simulink model "ebm_2022"  (R2022a)
settings: Solver=ode4  StartTime=0.0  StopTime=Inf  FixedStep=0.1  RelTol=1e-3  EnableMultiTasking=on
PreLoadFcn:
  | initialize;
values from neighbouring files (symbols this model uses):
  offset = 100.0*(mean(T_ambient) - mean(T_heater))    [initialize.m]
libraries: arduinolib x4, dspstat3 x2
PostSaveFcn:
  | initialize;
settings Model: ExtModeTrigDuration=2  Creator=user  LastModifiedBy=manur
settings SolverCC: AlgebraicLoopSolver=TrustRegion  AutoInsertRateTranBlk=on
settings DataIOCC: ReturnWorkspaceOutputs=off
settings OptimizationCC: EnhancedBackFolding=on  PassReuseOutputArgsAs=Individual arguments  MaxStackSize=64  OptimizeBlockOrder=speed  DifferentSizesBufferReuse=on  OptimizationCustomize=off  EfficientTunableParamExpr=on
settings DebuggingCC: ParameterTunabilityLossMsg=error  UnconnectedInputMsg=warning  UnconnectedOutputMsg=warning  UnconnectedLineMsg=warning  SFMachineParentedDataDiag=warning  ArithmeticOperatorsInVariantConditions=warning
settings HardwareCC: ProdBitPerInt=16  ProdBitPerPointer=16  ProdBitPerSizeT=16  ProdBitPerPtrDiffT=16  ProdLargestAtomicFloat=None  ProdWordSize=8  ProdHWDeviceType=Atmel->AVR
settings SFSimCC: SimUseLocalCustomCode=off  MATLABDynamicMemAlloc=off  CustomCodeUndefinedFunction=UseInterfaceOnly
settings SFSimCC: SimCustomInitializer=|
  | analogWrite(9, 255); // the fan has quite significant stiction friction, so we start with a full speed!
  | delay(10);
settings SFSimCC: SimCustomTerminator=|
  | analogWrite(9, 0);
  | analogWrite(10, 0);
  | delay(1);
settings RTWCC: SystemTargetFile=ert.tlc  HardwareBoard=Arduino Uno  TemplateMakefile=ert_default_tmf  GenerateReport=on  RTWUseLocalCustomCode=off  Toolchain=Arduino AVR  BuildConfiguration=Faster Runs  IncludeHyperlinkInReport=on  LaunchReport=on  GenerateTraceInfo=on  GenerateTraceReport=on  GenerateTraceReportSl=on  GenerateTraceReportSf=on  GenerateTraceReportEml=on  DLArmComputeVersion=19.05
settings CodeAppCC: ForceParamTrailComments=on  IgnoreCustomStorageClasses=off  OperatorAnnotations=on  SimulinkDataObjDesc=on  SFDataObjDesc=on  InsertBlockDesc=on
settings ERTTargetCC: SupportContinuousTime=on  SupportVariableSizeSignals=on  ExtMode=on  ExtModeMexArgs='127.0.0.1' 0 17725

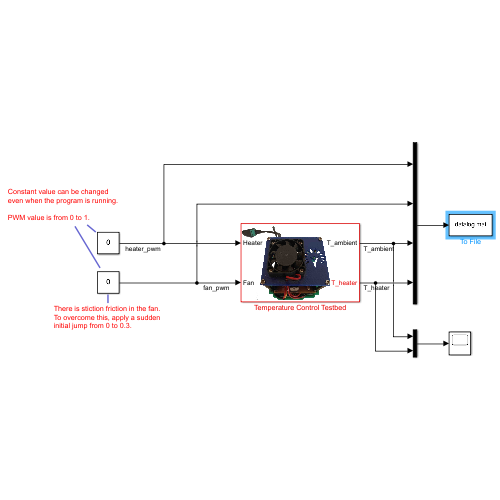
[thumbnail: Simulink's stored preview of the top-level diagram]
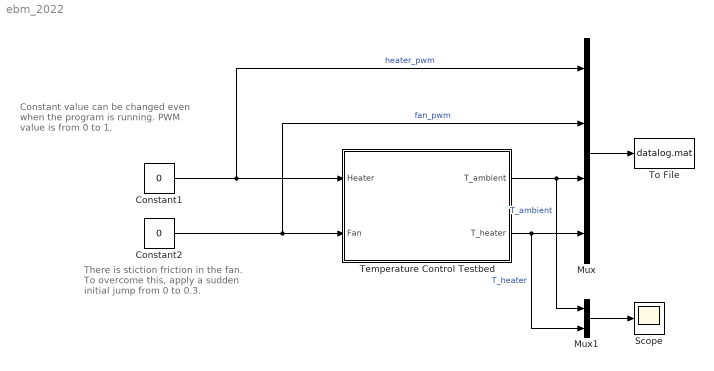
== system ebm_2022 ==
  note: There is stiction friction in the fan.
      | To overcome this, apply a sudden
      | initial jump from 0 to 0.3.
  note: Constant value can be changed
      | even when the program is running.
      |
      | PWM value is from 0 to 1.
  Constant1 : Constant  Value=0
  Constant2 : Constant  Value=0
  Mux : Mux
  Mux1 : Mux  Inputs=2
  Scope : Scope
  Temperature Control Testbed : Subsystem
      mask Display: image('$imagefile'); % Use "Edit Image" on toolstrip to change.
  To File : ToFile  Filename=datalog.mat  MatrixName=datalog
  wires:
  Constant1/1 -> Mux/1, Temperature Control Testbed/1(Heater)  "heater_pwm"
  Constant2/1 -> Mux/2, Temperature Control Testbed/2(Fan)  "fan_pwm"
  Temperature Control Testbed/2(T_heater) -> Mux1/2, Mux/4  "T_heater"
  Temperature Control Testbed/1(T_ambient) -> Mux1/1, Mux/3  "T_ambient"
  Mux/1 -> To File/1
  Mux1/1 -> Scope/1

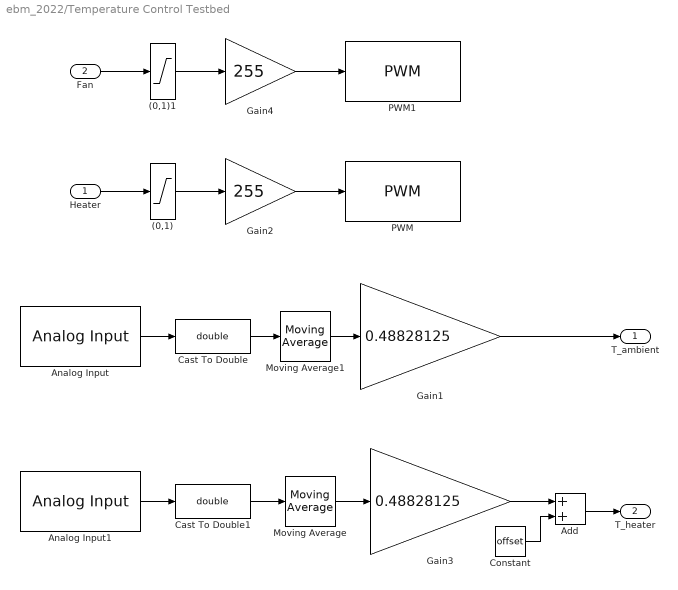
== system ebm_2022/Temperature Control Testbed ==
  Heater : Inport
  Fan : Inport  Port=2
  (0,1) : Saturate  UpperLimit=1  LowerLimit=0
  (0,1)1 : Saturate  UpperLimit=1  LowerLimit=0
  Add : Sum
  Analog Input : arduinolib/Analog Input  pinNumber=0  ReadResultsOnly=off  ConversionTriggerSource=Software  ExternalTriggerType=uint32(0)  OutputDataType=uint16  EnableConversionCompleteNotify=off  EnableOuputStatus=off  SampleTime=0.1  blockPlatform=arduino
  Analog Input1 : arduinolib/Analog Input  pinNumber=1  ReadResultsOnly=off  ConversionTriggerSource=Software  ExternalTriggerType=uint32(0)  OutputDataType=uint16  EnableConversionCompleteNotify=off  EnableOuputStatus=off  SampleTime=0.1  blockPlatform=arduino
  Cast To Double : DataTypeConversion  OutDataTypeStr=double  SaturateOnIntegerOverflow=off  RndMeth=Floor
  Cast To Double1 : DataTypeConversion  OutDataTypeStr=double  SaturateOnIntegerOverflow=off  RndMeth=Floor
  Constant : Constant  Value=offset
  Gain1 : Gain  Gain=0.48828125
  Gain2 : Gain  Gain=255
  Gain3 : Gain  Gain=0.48828125
  Gain4 : Gain  Gain=255
  Moving Average : dspstat3/Moving Average  Method=Sliding window  ForgettingFactorPort=off  SpecifyWindowLength=on  WindowLength=4  ForgettingFactor=0.9  SimulateUsing=Code generation
  Moving Average1 : dspstat3/Moving Average  Method=Sliding window  ForgettingFactorPort=off  SpecifyWindowLength=on  WindowLength=4  ForgettingFactor=0.9  SimulateUsing=Code generation
  PWM : arduinolib/PWM  pinNumber=10  frequencyType=Default  desiredFrequency=20000  achievableFrequency=20000
  PWM1 : arduinolib/PWM  pinNumber=9  frequencyType=Default  desiredFrequency=20000  achievableFrequency=20000
  T_ambient : Outport  VectorParamsAs1DForOutWhenUnconnected=off
  T_heater : Outport  Port=2  VectorParamsAs1DForOutWhenUnconnected=off
  wires:
  Gain2/1 -> PWM/1
  Analog Input/1 -> Cast To Double/1
  Cast To Double/1 -> Moving Average1/1
  Cast To Double1/1 -> Moving Average/1
  Analog Input1/1 -> Cast To Double1/1
  Gain4/1 -> PWM1/1
  Fan/1 -> (0,1)1/1
  Heater/1 -> (0,1)/1
  (0,1)1/1 -> Gain4/1
  (0,1)/1 -> Gain2/1
  Add/1 -> T_heater/1
  Constant/1 -> Add/2
  Gain1/1 -> T_ambient/1
  Gain3/1 -> Add/1
  Moving Average/1 -> Gain3/1
  Moving Average1/1 -> Gain1/1
